simulink model "MPC_Stabilization"  (R2020b)
settings: Solver=VariableStepAuto  StartTime=0.0  StopTime=40  RelTol=1e-3
PreLoadFcn:
  | run('MPC_Stabilization_Init.m')
InitFcn:
  | run('MPC_Stabilization_Init.m')
values from neighbouring files (symbols this model uses):
  A = state_space.A    [MPC_Stabilization_Init.m]
  B = state_space.B    [MPC_Stabilization_Init.m]
  C = state_space.C    [MPC_Stabilization_Init.m]
  F = (2*T_'*Q_*S_)'    [MPC_Stabilization_Init.m]
  G = [G;G_;-G_]    [MPC_Stabilization_Init.m]
  H = 2*(S_'*Q_*S_+ R_)    [MPC_Stabilization_Init.m]
  N = 10    [MPC_Stabilization_Init.m]
  S = [S; -s1; s1]    [MPC_Stabilization_Init.m]
  Ts = 1    [MPC_Stabilization_Init.m]
  W = [umax*ones(N,1);-umin*ones(N,1);ymax*ones(N,1);-ymin*ones(N,1)]    [MPC_Stabilization_Init.m]
  x_0 = [8 -5]'    [MPC_Stabilization_Init.m]
settings Model: Creator=hassan  LastModifiedBy=hassan

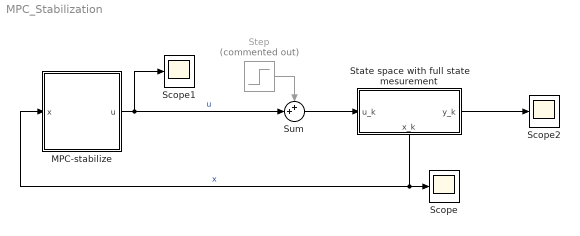
== system MPC_Stabilization ==
  MPC-stabilize : Subsystem  StartFcn=""  StopFcn=MPC_Stabilization_Init
  Scope : Scope
  Scope1 : Scope
  Scope2 : Scope
  State space with full state mesurement : Subsystem
      settings: PortSchema="{\"entries\":[{\"content\":{\"sides\":[{\"content\":{\"connectorIds\":[\"In1\"]},\"type\":\"ConnectorPlacement.EquallySpacedRectSide\",\"uuid\":\"af8233aa-8abb-4886-bf43-cd1df4b87fab\"},{\"content\":{\"connectorIds\":[\"Out1\"],\"side\":\"RIGHT\"},\"type\":\"ConnectorPlacement.EquallySpacedRectSide\",\"uuid\":\"f0184c17-054b-49be-872c-09bd334a5600\"},{\"content\":{\"connectorIds\":[],\"side\":\"TOP\"},\"type\":\"ConnectorPlacement.EquallySpacedRectSide\",\"uuid\":\"196756da-402b-4ddd-adb8-b38ddd7714c4\"},{\"content\":{\"connectorIds\":[\"Out2\"],\"side\":\"BOTTOM\"},\"type\":\"ConnectorPlacement.EquallySpacedRectSide\",\"uuid\":\"e01ecabc-bb09-404c-a3dc-123317d894ec\"},{\"content\":{\"connectorIds\":[],\"side\":\"HIDDEN\"},\"type\":\"ConnectorPlacement.EquallySpacedRectSide\",\"uuid\":\"74208052-37b1-4021-8931-49b821996a73\"}]},\"type\":\"ConnectorPlacement.EquallySpacedConnector\",\"uuid\":\"975ee949-398e-43e2-80ac-c4948e7e5efa\"}],\"packageUris\":[\"http://schema.mathworks.com/mf0/Connector/R2020b\"],\"version\":\"1.0\"}"
  Step : Step  Commented=on  Time=20  After=2  SampleTime=0
  Sum : Sum  Inputs=++|
  wires:
  State space with full state mesurement/2(x_k) -> MPC-stabilize/1(x), Scope/1  "x"
  MPC-stabilize/1(u) -> Sum/2, Scope1/1  "u"
  State space with full state mesurement/1(y_k) -> Scope2/1
  Sum/1 -> State space with full state mesurement/1(u_k)
  Step/1 -> Sum/1

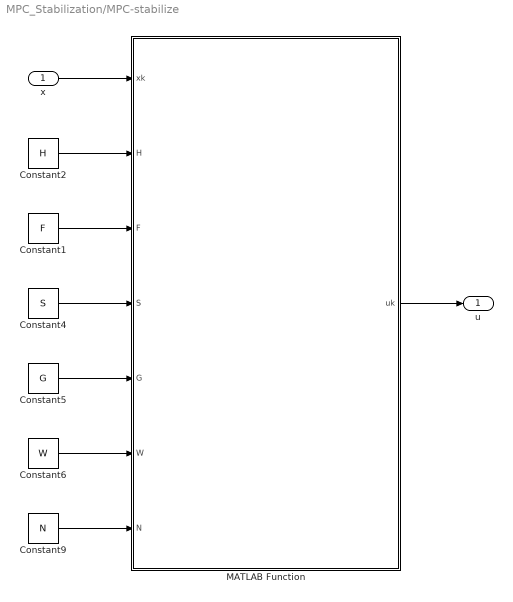
== system MPC_Stabilization/MPC-stabilize ==
  x : Inport
  Constant1 : Constant  Value=F
  Constant2 : Constant  Value=H
  Constant4 : Constant  Value=S
  Constant5 : Constant  Value=G
  Constant6 : Constant  Value=W
  Constant9 : Constant  Value=N
  MATLAB Function : MATLAB Function  TreatAsAtomicUnit=on
  u : Outport  VectorParamsAs1DForOutWhenUnconnected=off
  wires:
  x/1 -> MATLAB Function/1(xk)
  Constant2/1 -> MATLAB Function/2(H)
  Constant1/1 -> MATLAB Function/3(F)
  Constant4/1 -> MATLAB Function/4(S)
  Constant5/1 -> MATLAB Function/5(G)
  Constant6/1 -> MATLAB Function/6(W)
  Constant9/1 -> MATLAB Function/7(N)
  MATLAB Function/1(uk) -> u/1

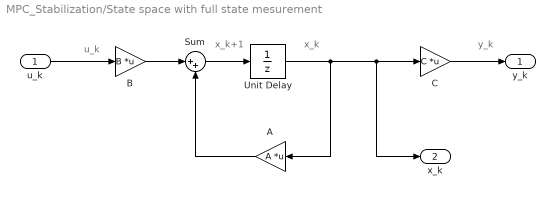
== system MPC_Stabilization/State space with full state mesurement ==
  note: x_k
  note: u_k
  note: x_k+1
  note: y_k
  u_k : Inport
  A : Gain  Gain=A  Multiplication=Matrix(K*u)
  B : Gain  Gain=B  Multiplication=Matrix(K*u)
  C : Gain  Gain=C  Multiplication=Matrix(K*u)
  Sum : Sum  Inputs=|++
  Unit Delay : UnitDelay  InitialCondition=x_0  SampleTime=Ts  HasFrameUpgradeWarning=on
  y_k : Outport  VectorParamsAs1DForOutWhenUnconnected=off
  x_k : Outport  Port=2  VectorParamsAs1DForOutWhenUnconnected=off
  wires:
  B/1 -> Sum/1
  A/1 -> Sum/2
  Sum/1 -> Unit Delay/1
  C/1 -> y_k/1
  u_k/1 -> B/1
  Unit Delay/1 -> A/1, x_k/1, C/1

== matlab function MPC_Stabilization/MPC-stabilize/MATLAB Function ==
  settings: updateMethod=DISCRETE  sampleTime=Ts
  data: xk input; uk output; H input; F input; S input; G input; W input; N input
function uk = MPC_Stabilisation(xk,H,F,S,G,W,N)

    %m =

    coder.extrinsic('optimoptions');
    coder.extrinsic('try');
    options = optimoptions('quadprog');
    options = optimoptions(options, 'Display', 'off');
    coder.extrinsic('quadprog');
    
    %Z = zeros(  );

    % sol = quadprog(,  ,  ,  , [], [], [], [], [], options);  
    
    if ~isempty(sol)
        Z = sol;
    else 
        error('QP Solver: QP problem infeasable, try relaxing constraints.');
    end

 
    % uk =
    

end
